simulink library "satelliteDynamics_lib"  (R2018b)
settings: Solver=VariableStepAuto  StartTime=0.0  StopTime=10.0  RelTol=1e-3
undefined symbols (not defined in the file or in its folder): DiscIntNeverNeededParam, fswParams, q_body, r_eci_km, simParams, v_eci_km, w_body_radps
libraries: vrlib x2, aerolibutil x1, sharedutil x1, state_bus x1
settings Model: Creator=colem  LastModifiedBy=colem

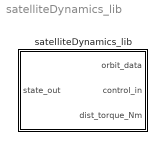
== system satelliteDynamics_lib ==
  satelliteDynamics_lib : Subsystem

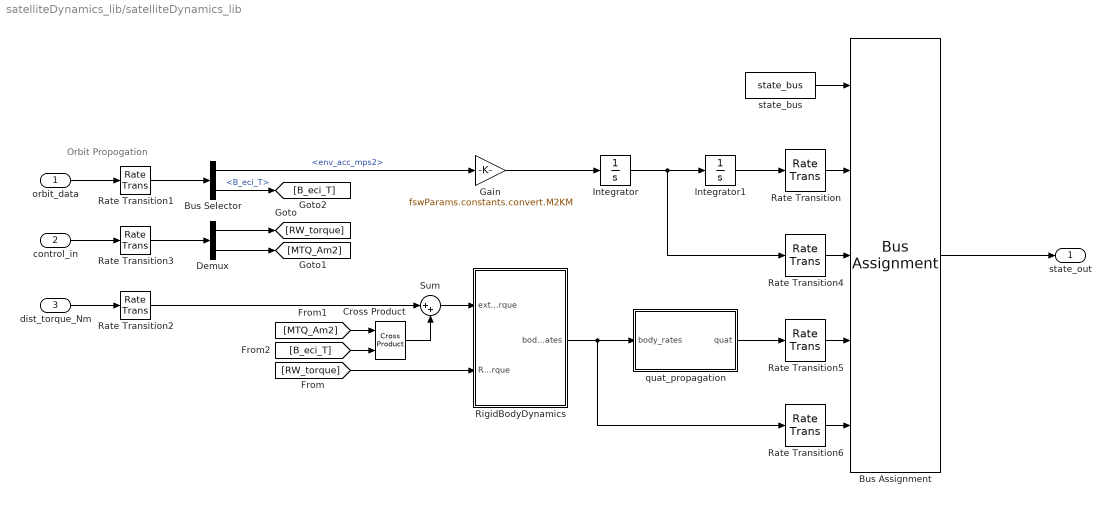
== system satelliteDynamics_lib/satelliteDynamics_lib ==
  note: Orbit Propogation
  orbit_data : Inport
  control_in : Inport  Port=2
  dist_torque_Nm : Inport  Port=3
  Bus Assignment : BusAssignment  AssignedSignals=r_eci_km,v_eci_km,q_body,w_body_radps
  Bus Selector : BusSelector  OutputSignals=env_acc_mps2,B_eci_T
  Cross Product : vrlib/Utilities/Cross Product
      settings: SourceProductBaseCode=VR
  Demux : Demux  Outputs=[3 3]
  Gain : Gain  Gain=fswParams.constants.convert.M2KM
  Integrator : Integrator  InitialCondition=simParams.initialConditions.v0
  Integrator1 : Integrator  InitialCondition=simParams.initialConditions.r0
  Rate Transition : RateTransition  InitialCondition=simParams.initialConditions.r0
  Rate Transition1 : RateTransition  OutPortSampleTime=simParams.sample_time_s
  Rate Transition2 : RateTransition  OutPortSampleTime=simParams.sample_time_s
  Rate Transition3 : RateTransition  OutPortSampleTime=simParams.sample_time_s
  Rate Transition4 : RateTransition  InitialCondition=simParams.initialConditions.v0
  Rate Transition5 : RateTransition  InitialCondition=simParams.initialConditions.q0
  Rate Transition6 : RateTransition  InitialCondition=simParams.initialConditions.w0
  RigidBodyDynamics : Subsystem
  Sum : Sum  Inputs=|++
  quat_propagation : Subsystem
  state_bus : state_bus/state_bus  SystemSampleTime=-1
  state_out : Outport
  wires:
  Cross Product/1 -> Sum/2
  [B_eci_T] -> Cross Product/2
  Bus Selector/2 -> [B_eci_T]  "<B_eci_T>"
  Rate Transition1/1 -> Bus Selector/1
  Bus Selector/1 -> Gain/1  "<env_acc_mps2>"
  orbit_data/1 -> Rate Transition1/1
  control_in/1 -> Rate Transition3/1
  Integrator/1 -> Rate Transition4/1, Integrator1/1
  Integrator1/1 -> Rate Transition/1
  Gain/1 -> Integrator/1
  Bus Assignment/1 -> state_out/1
  dist_torque_Nm/1 -> Rate Transition2/1
  quat_propagation/1(quat) -> Rate Transition5/1
  RigidBodyDynamics/1(body_rates) -> Rate Transition6/1, quat_propagation/1(body_rates)
  Rate Transition2/1 -> Sum/1
  Rate Transition3/1 -> Demux/1
  Demux/1 -> [RW_torque]
  Demux/2 -> [MTQ_Am2]
  [RW_torque] -> RigidBodyDynamics/2(RW_torque)
  [MTQ_Am2] -> Cross Product/1
  Sum/1 -> RigidBodyDynamics/1(external_torque)
  state_bus/1 -> Bus Assignment/1
  Rate Transition/1 -> Bus Assignment/2
  Rate Transition4/1 -> Bus Assignment/3
  Rate Transition5/1 -> Bus Assignment/4
  Rate Transition6/1 -> Bus Assignment/5

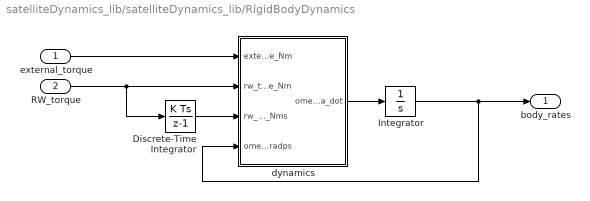
== system satelliteDynamics_lib/satelliteDynamics_lib/RigidBodyDynamics ==
  external_torque : Inport
  RW_torque : Inport  Port=2
  Discrete-Time Integrator : DiscreteIntegrator  InitialCondition=[0;0;0]  SampleTime=-1  ICPrevOutput=DiscIntNeverNeededParam  ICPrevScaledInput=DiscIntNeverNeededParam
  Integrator : Integrator  InitialCondition=simParams.initialConditions.w0
  dynamics : Subsystem
  body_rates : Outport
  wires:
  RW_torque/1 -> dynamics/2(rw_torque_Nm), Discrete-Time Integrator/1
  Discrete-Time Integrator/1 -> dynamics/3(rw_momentum_Nms)
  Integrator/1 -> body_rates/1, dynamics/4(omega_radps)
  external_torque/1 -> dynamics/1(external_torque_Nm)
  dynamics/1(omega_dot) -> Integrator/1

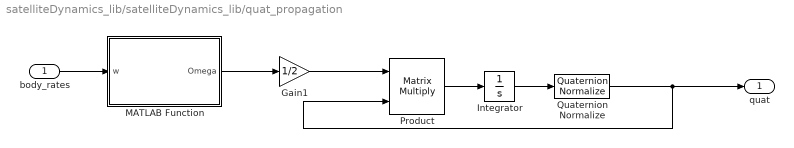
== system satelliteDynamics_lib/satelliteDynamics_lib/quat_propagation ==
  body_rates : Inport
  Gain1 : Gain  Gain=1/2
  Integrator : Integrator  InitialCondition=simParams.initialConditions.q0
  MATLAB Function : MATLAB Function  TreatAsAtomicUnit=on
  Product : Product  Multiplication=Matrix(*)  RndMeth=Zero
  Quaternion Normalize : sharedutil/Quaternion Normalize  aMode=aMode
      settings: SourceProductName=Aerospace Blockset  SourceProductBaseCode=AE
  quat : Outport
  wires:
  Product/1 -> Integrator/1
  Integrator/1 -> Quaternion Normalize/1
  Gain1/1 -> Product/1
  Quaternion Normalize/1 -> quat/1, Product/2
  body_rates/1 -> MATLAB Function/1(w)
  MATLAB Function/1(Omega) -> Gain1/1

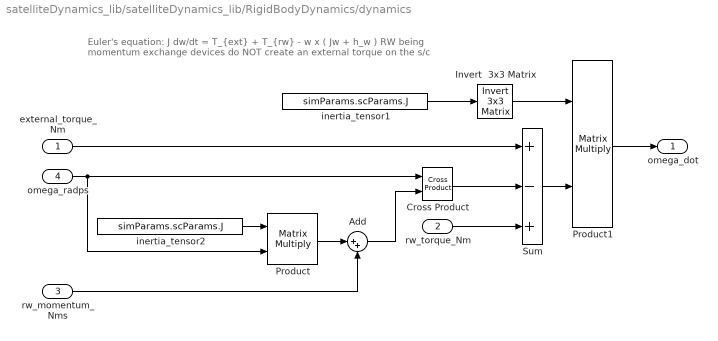
== system satelliteDynamics_lib/satelliteDynamics_lib/RigidBodyDynamics/dynamics ==
  note: Euler's equation: J dw/dt = T_{ext} + T_{rw} - w x ( Jw + h_w )
      |
      | RW being momentum exchange devices do NOT create
      | an external torque on the s/c
  external_torque_Nm : Inport
  rw_torque_Nm : Inport  Port=2
  rw_momentum_Nms : Inport  Port=3
  omega_radps : Inport  Port=4
  Add : Sum  Inputs=|++
  Cross Product : vrlib/Utilities/Cross Product
      settings: SourceProductBaseCode=VR
  Invert  3x3 Matrix : aerolibutil/Invert  3x3 Matrix
  Product : Product  Multiplication=Matrix(*)  RndMeth=Zero
  Product1 : Product  Multiplication=Matrix(*)  RndMeth=Zero
  Sum : Sum  Inputs=+-+
  inertia_tensor1 : Constant  Value=simParams.scParams.J
  inertia_tensor2 : Constant  Value=simParams.scParams.J
  omega_dot : Outport
  wires:
  rw_torque_Nm/1 -> Sum/3
  Add/1 -> Cross Product/2
  Product/1 -> Add/1
  Cross Product/1 -> Sum/2
  inertia_tensor1/1 -> Invert  3x3 Matrix/1
  Invert  3x3 Matrix/1 -> Product1/1
  Product1/1 -> omega_dot/1
  Sum/1 -> Product1/2
  inertia_tensor2/1 -> Product/1
  omega_radps/1 -> Cross Product/1, Product/2
  external_torque_Nm/1 -> Sum/1
  rw_momentum_Nms/1 -> Add/2

== matlab function satelliteDynamics_lib/quat_propagation/MATLAB Function ==
  data: w input; Omega output
function Omega = skew_sym(w)
%#codegen

    w_skew = ...
        [0 w(3) -w(2);
        -w(3) 0 w(1);
        w(2) -w(1) 0];

    Omega = ...
        [0 -w';
        w w_skew];
